simulink model "Merged_Model"  (R2020b)
settings: Solver=ode4  StartTime=0  StopTime=5000  FixedStep=0.1  MaxStep=0.1  RelTol=1e-3  EnableMultiTasking=on
values from neighbouring files (symbols this model uses):
  A_mem = 7.4    [ptoSimInputFile.m]
  A_p = V_tank_i / L_tank    (= 0.8420608)    [ptoSimInputFile.m]
  A_w = 5.56e-12    [ptoSimInputFile.m]
  angVelInit = n_shaft_ref_m    (= 50)    [ptoSimInputFile.m]
  b = b_prime / 1e3 * 1e3 * rho_f    (= 81215.9231426)    [ptoSimInputFile.m]
  C_f_i = 35    [ptoSimInputFile.m]
  D = 1.47e-9    (= 1.47e-09)    [ptoSimInputFile.m]
  eta_cp = 0.65    [ptoSimInputFile.m]
  eta_hp = 0.85    [ptoSimInputFile.m]
  eta_motor = .95    (= 0.95)    [ptoSimInputFile.m]
  J = 20*100    (= 2000)    [ptoSimInputFile.m]
  Kd = Kp*100    (= 0.001)    [ptoSimInputFile.m]
  Kd_k = Kp_k*100    (= -6.66666666667e-12)    [ptoSimInputFile.m]
  Ki = 0    [ptoSimInputFile.m]
  Ki_k = 0    [ptoSimInputFile.m]
  Kp = 1e-5    (= 1e-05)    [ptoSimInputFile.m]
  Kp_k = (-1e-13)/1.5    (= -6.66666666667e-14)    [ptoSimInputFile.m]
  L_mem = .96    (= 0.96)    [ptoSimInputFile.m]
  L_tank = 1    [ptoSimInputFile.m]
  n_par = 320    [ptoSimInputFile.m]
  n_ser = 1    [ptoSimInputFile.m]
  n_shaft_ref_m = 50    [ptoSimInputFile.m]
  nu = 8.56e-7    (= 8.56e-07)    [ptoSimInputFile.m]
  num_batches = 10*tFactor    (= 10)    [ptoSimInputFile.m]
  Omega_1_init = Q_1_init/(0.7*sqrt(2*p_h_init/rho_f))    [ptoSimInputFile.m]
  Omega_2_init = Q_2_init/(0.7*sqrt(2*p_c_init/rho_f))    [ptoSimInputFile.m]
  p_precharge = 0.9*p_lower_limit    (= 9600000)    [ptoSimInputFile.m]
  p_rated = 16e6    (= 16000000)    [ptoSimInputFile.m]
  ptosim = ptoSimClass('Non-Compressible Fluid Hydraulic')    [ptoSimInputFile.m]
  Q_cp = Q_p_des / RR_inst_des - Q_p_des    (= 0.17752896)    [ptoSimInputFile.m]
  rho_f = 1025    [ptoSimInputFile.m]
  Sc = nu/D    (= 582.31292517)    [ptoSimInputFile.m]
  thick = 7.112e-4    (= 0.0007112)    [ptoSimInputFile.m]
  V_0 = 6    [ptoSimInputFile.m]
  V_D_hpp = Q_p_des/n_shaft_ref_m    (= 0.0003945088)    [ptoSimInputFile.m]
  V_D_m = Q_2_des/n_shaft_ref_m    (= 0.000224)    [ptoSimInputFile.m]
  V_mem = A_mem * thick / 2    (= 0.00263144)    [ptoSimInputFile.m]
  V_rated = V_0*(1-(p_precharge/p_rated)^(1/1.4))    (= 1.83430127072)    [ptoSimInputFile.m]
  V_tank_i = (V_mem * n_ser * n_par * RR_tot)/(1 - RR_tot)    (= 0.8420608)    [ptoSimInputFile.m]
undefined symbols (not defined in the file or in its folder): body, constraint, pto
libraries: WECSim_Lib x5, dspswit3 x1
settings Model: Creator=mlawson  LastModifiedBy=Hayden
settings SolverCC: ZeroCrossControl=DisableAll  AlgebraicLoopSolver=LineSearch  AutoInsertRateTranBlk=on
settings DataIOCC: SaveFormat=Array  SaveOutput=off  SaveTime=off  ReturnWorkspaceOutputs=off
settings OptimizationCC: LifeSpan=inf  SimCompilerOptimization=on
settings DebuggingCC: UnderspecifiedInitializationDetection=Classic  MergeDetectMultiDrivingBlocksExec=none  SolverPrmCheckMsg=warning  AllowSymbolicDim=off  StateNameClashWarn=warning  SFUnexpectedBacktrackingDiag=warning  SFNoUnconditionalDefaultTransitionDiag=warning  ArithmeticOperatorsInVariantConditions=warning
settings HardwareCC: ProdBitPerPointer=32  ProdBitPerSizeT=32  ProdBitPerPtrDiffT=32  ProdLargestAtomicFloat=None  ProdIntDivRoundTo=Undefined  ProdEndianess=Unspecified  ProdWordSize=32  ProdHWDeviceType=32-bit Generic
settings ModelReferenceCC: PropagateSignalLabelsOutOfModel=off
settings SFSimCC: SimUseLocalCustomCode=off  CustomCodeUndefinedFunction=UseInterfaceOnly
settings RTWCC: RTWUseLocalCustomCode=off
settings CodeAppCC: StateflowObjectComments=on
settings GRTTargetCC: TargetLangStandard=C89/C90 (ANSI)
settings ConfigComp: CovMetricSettings=dw  CovSaveCumulativeToWorkspaceVar=on  CovSaveSingleToWorkspaceVar=on  CovExternalEMLEnable=off  CovSFcnEnable=off
settings SimscapeCC: SimscapeNormalizeSystem=off
settings ConfigurationSet: Description=SimMechanics 2G
settings ExplorerConfigSet: SimMechanicsOpenEditorOnUpdate=off  InternalSimMechanicsExplorerSettings="<ExplorerConfiguration><canonicalview>default</canonicalview><TilePanel><TileInfo><Tiles Columns=\"1\" Count=\"1\" Rows=\"1\"><Column Left=\"2\" Weight=\"1\"/><Column Left=\"1335\"/><Row Top=\"2\" Weight=\"1\"/><Row Top=\"911\"/><Tile Height=\"1\" Width=\"1\" X=\"0\" Y=\"0\"/></Tiles></TileInfo><SceneInfo><SceneViewer><BGColor><R>0.60000002384185791</R><G>0.60000002384185791</G><B>0.60000002384185791</B></BGColor><Camera><Position><X>365.37645888990272</X><Y>-369.82486814446582</Y><Z>359.64809521743916</Z></Position><Center><X>-6.7351450971904585</X><Y>2.2867358426280204</Y><Z>-12.463508769654169</Z></Center><Up><X>-0.40824829046386307</X><Y>0.40824829046386307</Y><Z>0.81649658092772615</Z></Up><Left>-57.820127362122818</Left><Right>57.820127362122818</Right><Bottom>-38.308817187253304</Bottom><Top>38.308817187253304</Top></Camera></SceneViewer></SceneInfo></TilePanel></ExplorerConfiguration>"

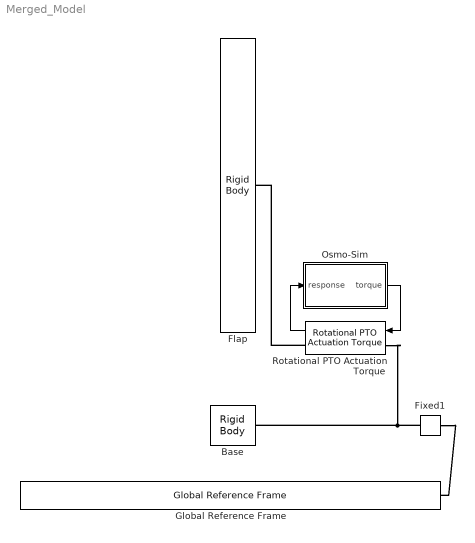
== system Merged_Model ==
  Base : WECSim_Lib/Body Elements/Rigid Body  body=body(2)
      settings: AttributesFormatString=%<body>  SourceProductName=WEC-Sim
  Fixed1 : WECSim_Lib/Constraints/Fixed  constraint=constraint(1)
      settings: AttributesFormatString=%<constraint>  SourceProductName=WEC-Sim
  Flap : WECSim_Lib/Body Elements/Rigid Body  body=body(1)
      settings: AttributesFormatString=%<body>  SourceProductName=WEC-Sim
  Global Reference Frame : WECSim_Lib/Frames/Global Reference Frame  waves=waves  simu=simu
      settings: SourceProductName=WEC-Sim
  Osmo-Sim : Subsystem
  Rotational PTO Actuation Torque : WECSim_Lib/PTOs/Rotational PTO Actuation Torque  pto=pto(1)
      settings: AttributesFormatString=%<pto>  SourceProductName=WEC-Sim
  wires:
  Rotational PTO Actuation Torque/1 -> Osmo-Sim/1(response)
  Osmo-Sim/1(torque) -> Rotational PTO Actuation Torque/1
  connections:
  Fixed1/LConn1 -- Global Reference Frame/RConn1
  Fixed1/RConn1 -- Rotational PTO Actuation Torque/LConn1 -- Base/RConn1
  Rotational PTO Actuation Torque/RConn1 -- Flap/RConn1

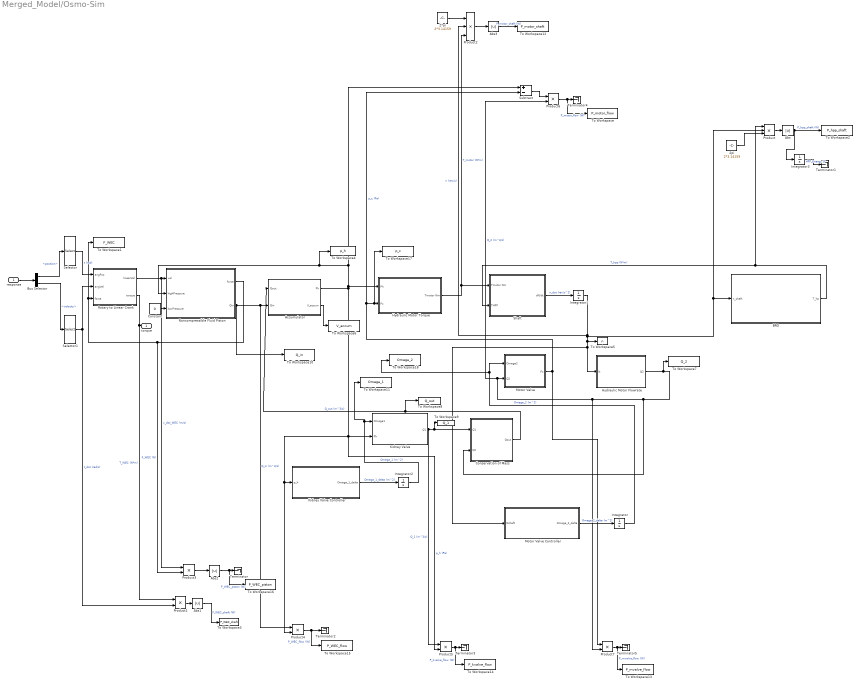
== system Merged_Model/Osmo-Sim ==
  response : Inport
  2*pi : Constant  Value=2*3.14159
  2pi : Constant  Value=2*3.14159  OutDataTypeStr=Inherit: Inherit via back propagation
  Abs{,1..3} (4 alike) : Abs
  Accumulator : Subsystem
  BRO : Subsystem
  Bus Selector : BusSelector  OutputSignals=position,velocity
  Conservation of Mass : Subsystem
  Constant : Constant  Value=0
  Hydraulic Motor Flowrate : Subsystem
  Hydraulic Motor Torque : Subsystem
  Integrator : Integrator  InitialCondition=Omega_2_init
  Integrator1 : Integrator  InitialCondition=angVelInit
  Integrator2 : Integrator  InitialCondition=Omega_1_init
  Integrator3 : Integrator
  Kidney Valve : Subsystem
  Kidney Valve Controller : Subsystem
  Motor Valve : Subsystem
  Motor Valve Controller : Subsystem
  Noncompressible Fluid Piston : Subsystem  mask{ptosim=ptosim.pistonNCF(1)}
      mask prompts: ptosim "Piston Name:"
      mask init:
      | if exist ('ptosim','var')
      |     h = [gcb '/To Workspace'];
      |     responseName = ['pistonNCF' num2str(ptosim.number) '_out'];
      |     set_param(h,'VariableName',responseName);
      |     if ischar(ptosim.topA)==1 ...
      |       || ischar(ptosim.botA)==1
      |          error('One of the piston variables is undefined. For example, ptosim.pistonNCF.variableName')
      |     end
      | end
      | clear h responseName
  Product : Product  Inputs=3
  Product{1,3..7} (6 alike) : Product
  Product2 : Product  Inputs=3
  Rotary to Linear Crank : Subsystem  AncestorBlock=PTOSim_Lib/Motion Conversion/Rotary to Linear Crank  mask{ptosim=ptosim.motionMechanism(1)}
      mask prompts: ptosim "Crank Name:"
      mask init:
      | if exist('ptosim','var')
      |     h = [gcb '/To Workspace'];
      |     responseName = ['motionMechanism' num2str(ptosim.number) '_out'];
      |     set_param(h,'VariableName',responseName);
      |     if ischar(ptosim.crank)==1 ...
      |             || ischar(ptosim.rodLength)==1 ...
      |             || ischar(ptosim.offset)==1 ...
      |             error('One of the rotary to linear crank variables is undefined. For example, ptosim.motionMechanism.variableName')
      |     end
      | end
      | clear h responseName
  Selector : Selector  InputPortWidth=6  IndexOptions=Index vector (dialog)  Indices=5  OutputSizes=1
  Selector1 : Selector  InputPortWidth=6  IndexOptions=Index vector (dialog)  Indices=5  OutputSizes=1
  Shaft : Subsystem
  Subtract : Sum  Inputs=+-
  Terminator{,1..5} (6 alike) : Terminator
  To Workspace : ToWorkspace  VariableName=P_motor_flow  SaveFormat=Timeseries  SampleTime=-1
  To Workspace1 : ToWorkspace  VariableName=F_WEC  SaveFormat=Timeseries  SampleTime=-1
  To Workspace10 : ToWorkspace  VariableName=Q_in  SaveFormat=Timeseries  SampleTime=-1
  To Workspace11 : ToWorkspace  VariableName=Omega_1  SaveFormat=Timeseries  SampleTime=-1
  To Workspace12 : ToWorkspace  VariableName=P_motor_shaft  SaveFormat=Timeseries  SampleTime=-1
  To Workspace13 : ToWorkspace  VariableName=P_mvalve_flow  SaveFormat=Timeseries  SampleTime=-1
  To Workspace14 : ToWorkspace  VariableName=P_kvalve_flow  SaveFormat=Timeseries  SampleTime=-1
  To Workspace15 : ToWorkspace  VariableName=P_WEC_flow  SaveFormat=Timeseries  SampleTime=-1
  To Workspace16 : ToWorkspace  VariableName=P_WEC_piston  SaveFormat=Timeseries  SampleTime=-1
  To Workspace17 : ToWorkspace  VariableName=p_c  SaveFormat=Timeseries  SampleTime=-1
  To Workspace18 : ToWorkspace  VariableName=Omega_2  SaveFormat=Timeseries  SampleTime=-1
  To Workspace2 : ToWorkspace  VariableName=P_hpp_shaft  SaveFormat=Timeseries  SampleTime=-1
  To Workspace3 : ToWorkspace  VariableName=P_WEC_shaft  SaveFormat=Timeseries  SampleTime=-1
  To Workspace4 : ToWorkspace  VariableName=p_h  SaveFormat=Timeseries  SampleTime=-1
  To Workspace5 : ToWorkspace  VariableName=n  SaveFormat=Timeseries  SampleTime=-1
  To Workspace6 : ToWorkspace  VariableName=V_accum  SaveFormat=Timeseries  SampleTime=-1
  To Workspace7 : ToWorkspace  VariableName=Q_2  SaveFormat=Timeseries  SampleTime=-1
  To Workspace8 : ToWorkspace  VariableName=Q_out  SaveFormat=Timeseries  SampleTime=-1
  To Workspace9 : ToWorkspace  VariableName=Q_1  SaveFormat=Timeseries  SampleTime=-1
  torque : Outport  VectorParamsAs1DForOutWhenUnconnected=off
  wires:
  response/1 -> Bus Selector/1
  Bus Selector/1 -> Selector/1  "<position>"
  Bus Selector/2 -> Selector1/1  "<velocity>"
  Rotary to Linear Crank/2(torque) -> Product1/1, torque/1  "T_WEC (N*m)"
  Selector/1 -> Rotary to Linear Crank/1(angPos)  "t (rad)"
  Selector1/1 -> Rotary to Linear Crank/2(angVel), Product1/2  "t_dot (rad/s)"
  Rotary to Linear Crank/1(linearVel) -> Product3/1, Noncompressible Fluid Piston/1(vel)  "x_dot_WEC (m/s)"
  Noncompressible Fluid Piston/1(force) -> Product3/2, To Workspace1/1, Rotary to Linear Crank/3(force)  "F_WEC (N)"
  Constant/1 -> Noncompressible Fluid Piston/3(lowPressure)
  Accumulator/1(Ph) -> Subtract/1, Noncompressible Fluid Piston/2(highPressure), To Workspace4/1, Hydraulic Motor Torque/1(Ph), Product5/2, Product4/2, Kidney Valve Controller/1(p_h), Kidney Valve/2(Ph)  "p_h (Pa)"
  Noncompressible Fluid Piston/2(Qin) -> To Workspace10/1, Product4/1, Accumulator/2(Qin)  "Q_in (m^3/s)"
  Motor Valve/1(Pc) -> Subtract/2, To Workspace17/1, Hydraulic Motor Torque/2(Pc), Product7/1  "p_c (Pa)"
  BRO/1(T_hp) -> Shaft/2(THPP), Product/1  "T_hpp (N*m)"
  Hydraulic Motor Torque/1(Tmotor Nm) -> Shaft/1(Tmotor Nm), Product2/3  "T_motor (N*m)"
  Integrator1/1 -> BRO/1(n_shaft), Product/2, Hydraulic Motor Flowrate/1(N), Motor Valve Controller/1(Nshaft), To Workspace5/1, Product2/2  "n (rev/s)"
  Shaft/1(dN/dt) -> Integrator1/1  "n_dot (rev/s^2)"
  Kidney Valve/1(Q1) -> Product5/1, Conservation of Mass/1(Q1), To Workspace9/1  "Q_1 (m^3/s)"
  Conservation of Mass/1(Qout) -> To Workspace8/1, Accumulator/1(Qout)  "Q_out (m^3/s)"
  Product/1 -> Abs/1
  Product1/1 -> Abs1/1
  2pi/1 -> Product/3
  Abs/1 -> Integrator3/1, To Workspace2/1  "P_hpp_shaft (W)"
  Abs1/1 -> To Workspace3/1  "P_WEC_shaft (W)"
  Hydraulic Motor Flowrate/1(Q2) -> To Workspace7/1, Conservation of Mass/2(Q2), Product7/2, Motor Valve/2(Q2), Product6/2  "Q_2 (m^3/s)"
  Motor Valve Controller/1(Omega_2_delta) -> Integrator/1  "Omega_2_delta (m^2)"
  Integrator/1 -> To Workspace18/1, Motor Valve/1(Omega2)  "Omega_2 (m^2)"
  Accumulator/2(V_accum) -> To Workspace6/1
  Kidney Valve Controller/1(Omega_1_delta) -> Integrator2/1  "Omega_1_delta (m^2)"
  Integrator2/1 -> To Workspace11/1, Kidney Valve/1(Omega1)  "Omega_1 (m^2)"
  2*pi/1 -> Product2/1
  Product3/1 -> Abs2/1
  Abs2/1 -> To Workspace16/1, Terminator/1  "P_WEC_piston (W)"
  Integrator3/1 -> Terminator1/1  "HPP_Energy (J)"
  Product2/1 -> Abs3/1
  Abs3/1 -> To Workspace12/1  "P_motor_shaft (W)"
  Product4/1 -> To Workspace15/1, Terminator2/1  "P_WEC_flow (W)"
  Product5/1 -> To Workspace14/1, Terminator3/1  "P_kvalve_flow (W)"
  Subtract/1 -> Product6/1
  Product6/1 -> To Workspace/1, Terminator4/1  "P_motor_flow (W)"
  Product7/1 -> To Workspace13/1, Terminator5/1  "P_mvalve_flow (W)"

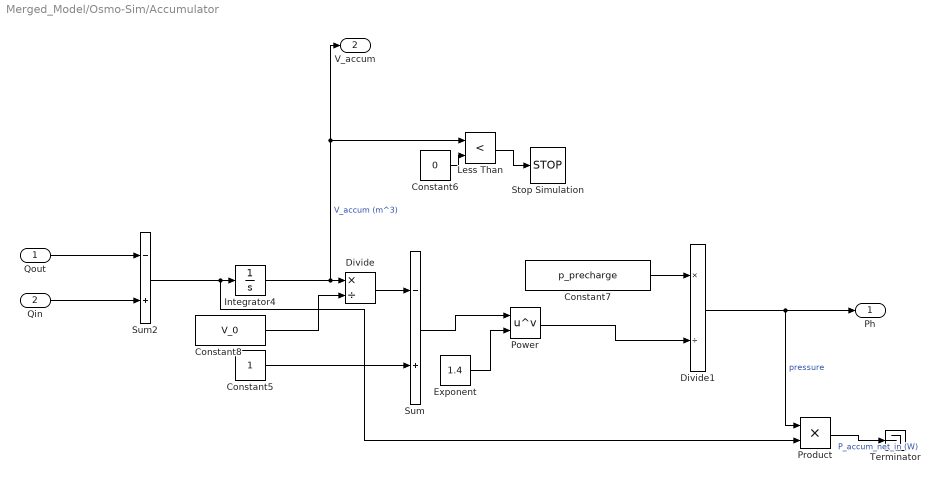
== system Merged_Model/Osmo-Sim/Accumulator ==
  Qout : Inport
  Qin : Inport  Port=2
  Constant5 : Constant
  Constant6 : Constant  Value=0
  Constant7 : Constant  Value=p_precharge
  Constant8 : Constant  Value=V_0
  Divide : Product  Inputs=*/
  Divide1 : Product  Inputs=*/
  Exponent : Constant  Value=1.4
  Integrator4 : Integrator  InitialCondition=V_rated
  Less Than : RelationalOperator  Operator=<  OutDataTypeStr=boolean  RndMeth=Simplest
  Power : Math  Operator=pow  SaturateOnIntegerOverflow=on
  Product : Product
  Stop Simulation : Stop
  Sum : Sum  Inputs=-+
  Sum2 : Sum  Inputs=-+
  Terminator : Terminator
  Ph : Outport
  V_accum : Outport  Port=2
  wires:
  Constant8/1 -> Divide/2
  Qout/1 -> Sum2/1
  Power/1 -> Divide1/2
  Less Than/1 -> Stop Simulation/1
  Integrator4/1 -> V_accum/1, Less Than/1, Divide/1  "V_accum (m^3)"
  Constant7/1 -> Divide1/1
  Divide1/1 -> Product/1, Ph/1  "pressure"
  Divide/1 -> Sum/1
  Constant5/1 -> Sum/2
  Qin/1 -> Sum2/2
  Constant6/1 -> Less Than/2
  Sum2/1 -> Product/2, Integrator4/1
  Exponent/1 -> Power/2
  Sum/1 -> Power/1
  Product/1 -> Terminator/1  "P_accum_net_in (W)"

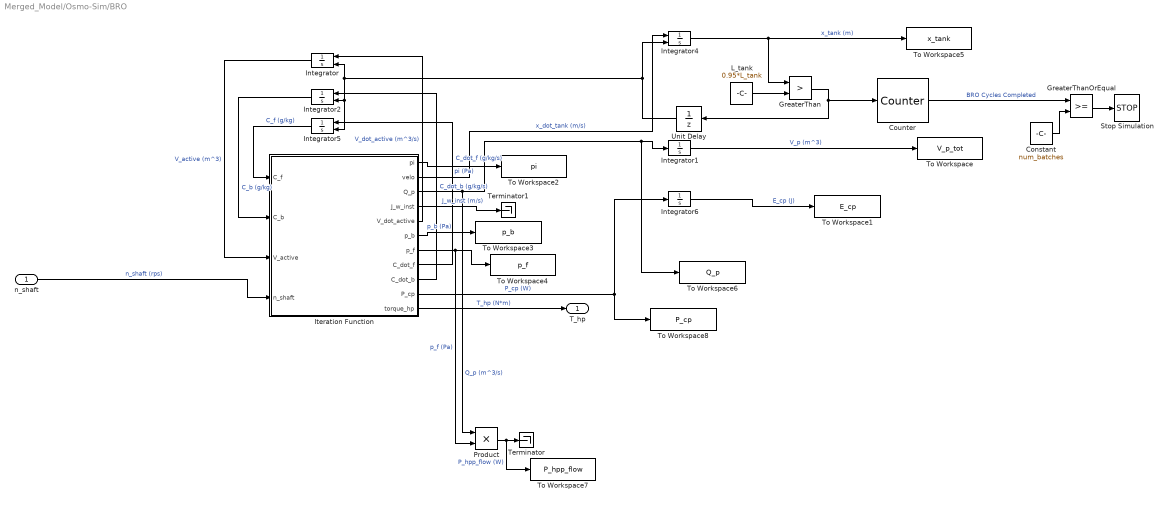
== system Merged_Model/Osmo-Sim/BRO ==
  n_shaft : Inport
  Constant : Constant  Value=num_batches
  Counter : dspswit3/Counter  Direction=Up  CountEvent=Rising edge  CounterSize=User defined  MaxCount=255  InitialCount=0  Output=Count  HitValue=32  ResetInput=off  SamplesPerFrame=1  Ts=1  CntDtype=double  HitDtype=Logical
  GreaterThan : RelationalOperator  Operator=>  OutDataTypeStr=boolean  RndMeth=Simplest
  GreaterThanOrEqual : RelationalOperator  OutDataTypeStr=boolean  RndMeth=Simplest
  Integrator : Integrator  ExternalReset=rising  InitialCondition=V_tank_i
  Integrator1 : Integrator
  Integrator2 : Integrator  ExternalReset=rising  InitialCondition=C_f_i
  Integrator4 : Integrator  ExternalReset=rising
  Integrator5 : Integrator  ExternalReset=rising  InitialCondition=C_f_i
  Integrator6 : Integrator
  Iteration Function : MATLAB Function  TreatAsAtomicUnit=on
  L_tank : Constant  Value=0.95*L_tank
  Product : Product
  Stop Simulation : Stop
  Terminator : Terminator
  Terminator1 : Terminator
  To Workspace : ToWorkspace  VariableName=V_p_tot  SaveFormat=Timeseries  SampleTime=-1
  To Workspace1 : ToWorkspace  VariableName=E_cp  SaveFormat=Timeseries  SampleTime=-1
  To Workspace2 : ToWorkspace  VariableName=pi  SaveFormat=Timeseries  SampleTime=-1
  To Workspace3 : ToWorkspace  VariableName=p_b  SaveFormat=Timeseries  SampleTime=-1
  To Workspace4 : ToWorkspace  VariableName=p_f  SaveFormat=Timeseries  SampleTime=-1
  To Workspace5 : ToWorkspace  VariableName=x_tank  SaveFormat=Timeseries  SampleTime=-1
  To Workspace6 : ToWorkspace  VariableName=Q_p  SaveFormat=Timeseries  SampleTime=-1
  To Workspace7 : ToWorkspace  VariableName=P_hpp_flow  SaveFormat=Timeseries  SampleTime=-1
  To Workspace8 : ToWorkspace  VariableName=P_cp  SaveFormat=Timeseries  SampleTime=-1
  Unit Delay : UnitDelay  SampleTime=-1  HasFrameUpgradeWarning=on
  T_hp : Outport
  wires:
  Integrator2/1 -> Iteration Function/2(C_b)  "C_b (g/kg)"
  Iteration Function/7(p_f) -> Product/2, To Workspace4/1  "p_f (Pa)"
  Iteration Function/5(V_dot_active) -> Integrator/1  "V_dot_active (m^3/s)"
  GreaterThan/1 -> Counter/1, Unit Delay/1
  Iteration Function/8(C_dot_f) -> Integrator5/1  "C_dot_f (g/kg/s)"
  Integrator1/1 -> To Workspace/1  "V_p (m^3)"
  L_tank/1 -> GreaterThan/2
  Integrator/1 -> Iteration Function/3(V_active)  "V_active (m^3)"
  Iteration Function/3(Q_p) -> To Workspace6/1, Integrator1/1, Product/1  "Q_p (m^3/s)"
  Iteration Function/9(C_dot_b) -> Integrator2/1  "C_dot_b (g/kg/s)"
  Integrator4/1 -> To Workspace5/1, GreaterThan/1  "x_tank (m)"
  Iteration Function/10(P_cp) -> Integrator6/1, To Workspace8/1  "P_cp (W)"
  Iteration Function/2(velo) -> Integrator4/1  "x_dot_tank (m/s)"
  Integrator5/1 -> Iteration Function/1(C_f)  "C_f (g/kg)"
  Iteration Function/6(p_b) -> To Workspace3/1  "p_b (Pa)"
  Iteration Function/4(J_w_inst) -> Terminator1/1  "J_w_inst (m/s)"
  Iteration Function/1(pi) -> To Workspace2/1  "pi (Pa)"
  Integrator6/1 -> To Workspace1/1  "E_cp (J)"
  Unit Delay/1 -> Integrator4/2, Integrator5/2, Integrator2/2, Integrator/2
  Counter/1 -> GreaterThanOrEqual/1  "BRO Cycles Completed"
  Constant/1 -> GreaterThanOrEqual/2
  GreaterThanOrEqual/1 -> Stop Simulation/1
  Iteration Function/11(torque_hp) -> T_hp/1  "T_hp (N*m)"
  n_shaft/1 -> Iteration Function/4(n_shaft)  "n_shaft (rps)"
  Product/1 -> To Workspace7/1, Terminator/1  "P_hpp_flow (W)"

== system Merged_Model/Osmo-Sim/Conservation of Mass ==
  Q1 : Inport
  Q2 : Inport  Port=2
  Add1 : Sum
  Qout : Outport
  wires:
  Add1/1 -> Qout/1
  Q2/1 -> Add1/1
  Q1/1 -> Add1/2

== system Merged_Model/Osmo-Sim/Hydraulic Motor Flowrate ==
  N : Inport
  Product2 : Product
  V_D_m : Constant  Value=V_D_m
  Q2 : Outport
  wires:
  Product2/1 -> Q2/1  "Q2"
  V_D_m/1 -> Product2/2
  N/1 -> Product2/1

== system Merged_Model/Osmo-Sim/Hydraulic Motor Torque ==
  Ph : Inport
  Pc : Inport  Port=2
  2pi : Constant  Value=2*3.14159
  Eta Motor : Constant  Value=eta_motor
  Product2 : Product  Inputs=***/
  Sum2 : Sum  Inputs=+-
  Vdm : Constant  Value=V_D_m
  Tmotor Nm : Outport
  wires:
  Eta Motor/1 -> Product2/3
  Ph/1 -> Sum2/1
  Product2/1 -> Tmotor Nm/1
  Vdm/1 -> Product2/2
  Sum2/1 -> Product2/1
  Pc/1 -> Sum2/2
  2pi/1 -> Product2/4

== system Merged_Model/Osmo-Sim/Kidney Valve ==
  note: Q1
  Omega1 : Inport
  Ph : Inport  Port=2
  Cf1 : Constant  Value=0.7
  Divide1 : Product  Inputs=***
  Divide2 : Product  Inputs=*/
  Gain1 : Gain  Gain=2
  Square Root1 : Sqrt  SaturateOnIntegerOverflow=on
  rho (kg/m^3) : Constant  Value=1025
  Q1 : Outport
  wires:
  Divide2/1 -> Square Root1/1
  Cf1/1 -> Divide1/1
  Square Root1/1 -> Divide1/3
  rho (kg/m^3)/1 -> Divide2/2
  Gain1/1 -> Divide2/1
  Divide1/1 -> Q1/1
  Ph/1 -> Gain1/1
  Omega1/1 -> Divide1/2

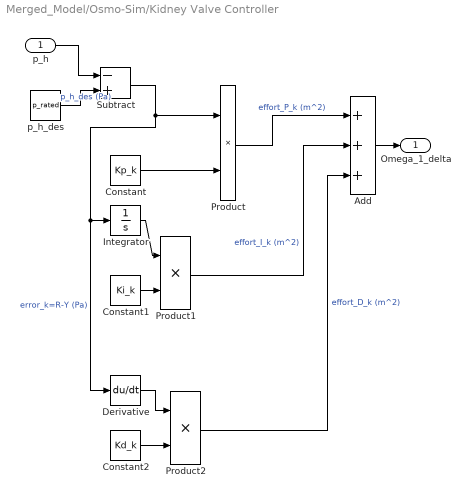
== system Merged_Model/Osmo-Sim/Kidney Valve Controller ==
  p_h : Inport
  Add : Sum  Inputs=+++
  Constant : Constant  Value=Kp_k
  Constant1 : Constant  Value=Ki_k
  Constant2 : Constant  Value=Kd_k
  Derivative : Derivative
  Integrator : Integrator
  Product : Product
  Product1 : Product
  Product2 : Product
  Subtract : Sum  Inputs=-+
  p_h_des : Constant  Value=p_rated
  Omega_1_delta : Outport
  wires:
  p_h/1 -> Subtract/1
  p_h_des/1 -> Subtract/2  "p_h_des (Pa)"
  Subtract/1 -> Product/1, Derivative/1, Integrator/1  "error_k=R-Y (Pa)"
  Integrator/1 -> Product1/1
  Constant1/1 -> Product1/2
  Constant/1 -> Product/2
  Product/1 -> Add/1  "effort_P_k (m^2)"
  Product1/1 -> Add/2  "effort_I_k (m^2)"
  Add/1 -> Omega_1_delta/1
  Constant2/1 -> Product2/2
  Derivative/1 -> Product2/1
  Product2/1 -> Add/3  "effort_D_k (m^2)"

== system Merged_Model/Osmo-Sim/Motor Valve ==
  Omega2 : Inport
  Q2 : Inport  Port=2
  Cf1 : Constant  Value=0.7
  Constant : Constant  Value=2
  Product : Product  Inputs=**/
  Product2 : Product  Inputs=*//
  Square : Math  Operator=square  SaturateOnIntegerOverflow=on
  rho (kg/m^3)1 : Constant  Value=1025
  Pc : Outport
  wires:
  Product/1 -> Pc/1
  Cf1/1 -> Product2/2
  Product2/1 -> Square/1
  Square/1 -> Product/1
  rho (kg/m^3)1/1 -> Product/2
  Constant/1 -> Product/3
  Omega2/1 -> Product2/3
  Q2/1 -> Product2/1

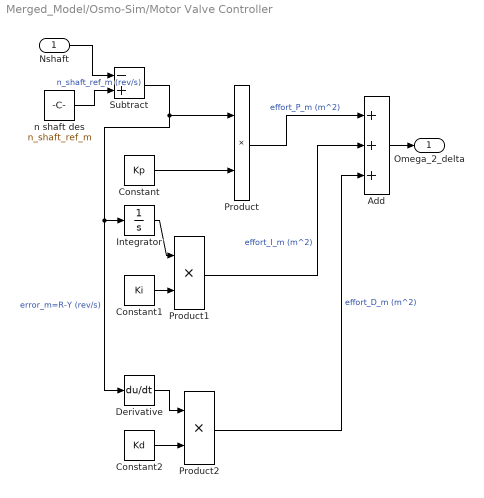
== system Merged_Model/Osmo-Sim/Motor Valve Controller ==
  Nshaft : Inport
  Add : Sum  Inputs=+++
  Constant : Constant  Value=Kp
  Constant1 : Constant  Value=Ki
  Constant2 : Constant  Value=Kd
  Derivative : Derivative
  Integrator : Integrator
  Product : Product
  Product1 : Product
  Product2 : Product
  Subtract : Sum  Inputs=-+
  n shaft des : Constant  Value=n_shaft_ref_m
  Omega_2_delta : Outport
  wires:
  Nshaft/1 -> Subtract/1
  n shaft des/1 -> Subtract/2  "n_shaft_ref_m (rev/s)"
  Subtract/1 -> Product/1, Derivative/1, Integrator/1  "error_m=R-Y (rev/s)"
  Integrator/1 -> Product1/1
  Constant1/1 -> Product1/2
  Constant/1 -> Product/2
  Product/1 -> Add/1  "effort_P_m (m^2)"
  Product1/1 -> Add/2  "effort_I_m (m^2)"
  Add/1 -> Omega_2_delta/1
  Constant2/1 -> Product2/2
  Derivative/1 -> Product2/1
  Product2/1 -> Add/3  "effort_D_m (m^2)"

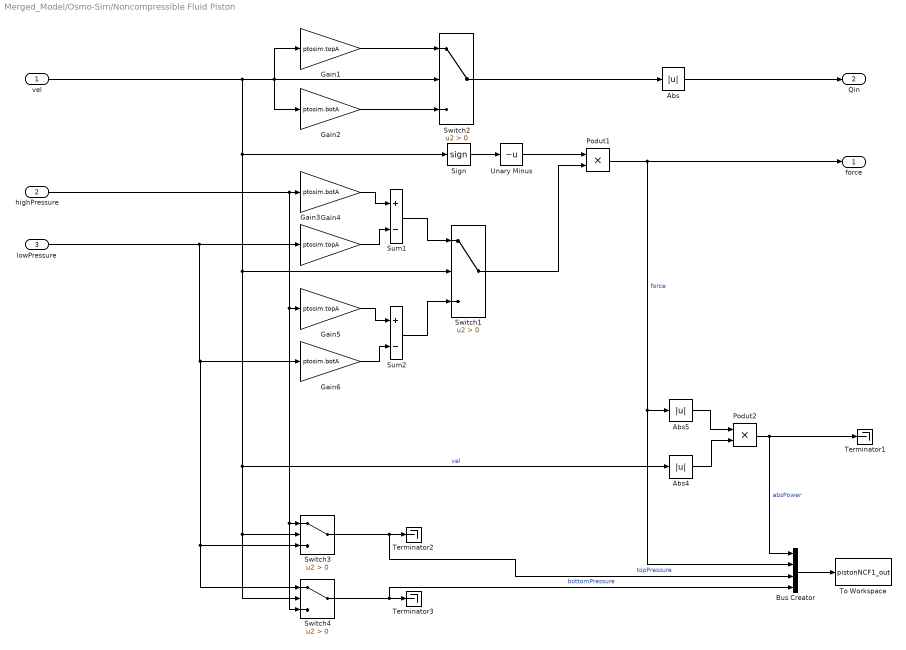
== system Merged_Model/Osmo-Sim/Noncompressible Fluid Piston ==
  vel : Inport
  highPressure : Inport  Port=2
  lowPressure : Inport  Port=3
  Abs : Abs
  Abs4 : Abs
  Abs5 : Abs
  Bus Creator : BusCreator  Inputs=4
  Gain1 : Gain  Gain=ptosim.topA
  Gain2 : Gain  Gain=ptosim.botA
  Gain3 : Gain  Gain=ptosim.topA
  Gain4 : Gain  Gain=ptosim.botA
  Gain5 : Gain  Gain=ptosim.topA
  Gain6 : Gain  Gain=ptosim.botA
  Podut1 : Product  RndMeth=Zero
  Podut2 : Product  RndMeth=Zero
  Sign : Signum
  Sum1 : Sum  Inputs=+-
  Sum2 : Sum  Inputs=+-
  Switch{1..4} (4 alike) : Switch  Criteria=u2 > Threshold
  Terminator1 : Terminator
  Terminator2 : Terminator
  Terminator3 : Terminator
  To Workspace : ToWorkspace  VariableName=pistonNCF1_out  SaveFormat=Structure With Time  SampleTime=-1
      settings: Decimation=round(simu.dtOut/simu.dt,0)
  Unary Minus : UnaryMinus
  force : Outport
  Qin : Outport  Port=2
  wires:
  Bus Creator/1 -> To Workspace/1
  Switch4/1 -> Terminator3/1, Bus Creator/4  "bottomPressure"
  Switch3/1 -> Terminator2/1, Bus Creator/3  "topPressure"
  Switch1/1 -> Podut1/2
  Unary Minus/1 -> Podut1/1
  Sign/1 -> Unary Minus/1
  Sum2/1 -> Switch1/3
  Gain6/1 -> Sum2/2
  Gain5/1 -> Sum2/1
  lowPressure/1 -> Gain3/1, Gain6/1, Switch3/3, Switch4/1
  Gain3/1 -> Sum1/2
  Gain4/1 -> Sum1/1
  Podut1/1 -> Abs5/1, Bus Creator/2, force/1  "force"
  Sum1/1 -> Switch1/1
  Gain2/1 -> Switch2/3
  Gain1/1 -> Switch2/1
  Abs4/1 -> Podut2/2
  Abs5/1 -> Podut2/1
  Podut2/1 -> Terminator1/1, Bus Creator/1  "absPower"
  vel/1 -> Gain1/1, Switch2/2, Gain2/1, Sign/1, Abs4/1, Switch3/2, Switch4/2, Switch1/2  "vel"
  highPressure/1 -> Gain5/1, Switch4/3, Switch3/1, Gain4/1
  Switch2/1 -> Abs/1
  Abs/1 -> Qin/1

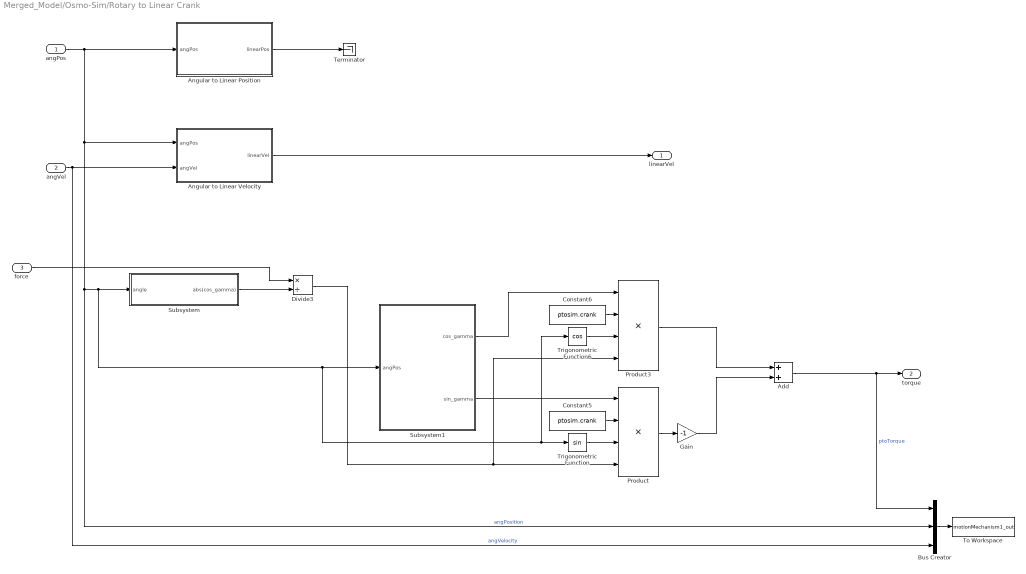
== system Merged_Model/Osmo-Sim/Rotary to Linear Crank ==
  angPos : Inport
  angVel : Inport  Port=2
  force : Inport  Port=3
  Add : Sum
  Angular to Linear Position : Subsystem
  Angular to Linear Velocity : Subsystem
  Bus Creator : BusCreator  Inputs=3
  Constant5 : Constant  Value=ptosim.crank
  Constant6 : Constant  Value=ptosim.crank
  Divide3 : Product  Inputs=*/
  Gain : Gain  Gain=-1
  Product : Product  Inputs=4
  Product3 : Product  Inputs=4
  Subsystem : Subsystem
  Subsystem1 : Subsystem  AncestorBlock=PTOSim_Lib/Motion Conversion/Rotary to Linear Adjustable Rod/Subsystem
  Terminator : Terminator
  To Workspace : ToWorkspace  VariableName=motionMechanism1_out  SaveFormat=Structure With Time  SampleTime=-1
      settings: Decimation=round(simu.dtOut/simu.dt,0)
  Trigonometric Function : Trigonometry
  Trigonometric Function6 : Trigonometry  Operator=cos
  linearVel : Outport
  torque : Outport  Port=2
  wires:
  Product/1 -> Gain/1
  Constant5/1 -> Product/2
  Trigonometric Function/1 -> Product/3
  angPos/1 -> Angular to Linear Position/1(angPos), Bus Creator/2, Subsystem/1(angle), Trigonometric Function6/1, Trigonometric Function/1, Subsystem1/1(angPos), Angular to Linear Velocity/1(angPos)  "angPosition"
  Subsystem1/2(sin_gamma) -> Product/1
  Product3/1 -> Add/1
  Gain/1 -> Add/2
  Divide3/1 -> Product3/4, Product/4
  Constant6/1 -> Product3/2
  Subsystem1/1(cos_gamma) -> Product3/1
  Trigonometric Function6/1 -> Product3/3
  force/1 -> Divide3/1
  Subsystem/1(abs(cos_gamma)) -> Divide3/2
  Bus Creator/1 -> To Workspace/1
  Add/1 -> torque/1, Bus Creator/1  "ptoTorque"
  Angular to Linear Velocity/1(linearVel) -> linearVel/1
  angVel/1 -> Angular to Linear Velocity/2(angVel), Bus Creator/3  "angVelocity"
  Angular to Linear Position/1(linearPos) -> Terminator/1

== system Merged_Model/Osmo-Sim/Shaft ==
  Tmotor Nm : Inport
  THPP : Inport  Port=2
  Constant4 : Constant  Value=2*pi
  Constant5 : Constant  Value=J
  Divide2 : Product  Inputs=*//
  Sum1 : Sum
  dN/dt : Outport
  wires:
  Constant4/1 -> Divide2/3
  Sum1/1 -> Divide2/1
  THPP/1 -> Sum1/2
  Constant5/1 -> Divide2/2
  Divide2/1 -> dN/dt/1  "dN/dt"
  Tmotor Nm/1 -> Sum1/1

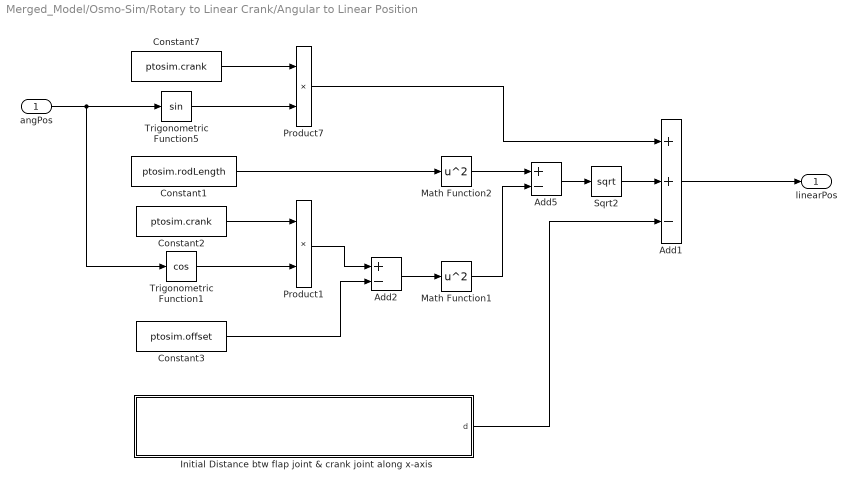
== system Merged_Model/Osmo-Sim/Rotary to Linear Crank/Angular to Linear Position ==
  angPos : Inport
  Add1 : Sum  Inputs=++-
  Add2 : Sum  Inputs=+-
  Add5 : Sum  Inputs=+-
  Constant1 : Constant  Value=ptosim.rodLength
  Constant2 : Constant  Value=ptosim.crank
  Constant3 : Constant  Value=ptosim.offset
  Constant7 : Constant  Value=ptosim.crank
  Initial Distance btw flap joint & crank joint along x-axis : Subsystem
  Math Function1 : Math  Operator=square  SignedPower=on  SaturateOnIntegerOverflow=on
  Math Function2 : Math  Operator=square  SignedPower=on  SaturateOnIntegerOverflow=on
  Product1 : Product  Inputs=**
  Product7 : Product  Inputs=**
  Sqrt2 : Sqrt  SaturateOnIntegerOverflow=on
  Trigonometric Function1 : Trigonometry  Operator=cos
  Trigonometric Function5 : Trigonometry
  linearPos : Outport
  wires:
  Math Function2/1 -> Add5/1
  Add1/1 -> linearPos/1
  Product7/1 -> Add1/1
  Sqrt2/1 -> Add1/2
  Math Function1/1 -> Add5/2
  Constant1/1 -> Math Function2/1
  Initial Distance btw flap joint & crank joint along x-axis/1(d) -> Add1/3
  Constant7/1 -> Product7/1
  Constant3/1 -> Add2/2
  Product1/1 -> Add2/1
  Trigonometric Function1/1 -> Product1/2
  Constant2/1 -> Product1/1
  Add5/1 -> Sqrt2/1
  Trigonometric Function5/1 -> Product7/2
  Add2/1 -> Math Function1/1
  angPos/1 -> Trigonometric Function5/1, Trigonometric Function1/1

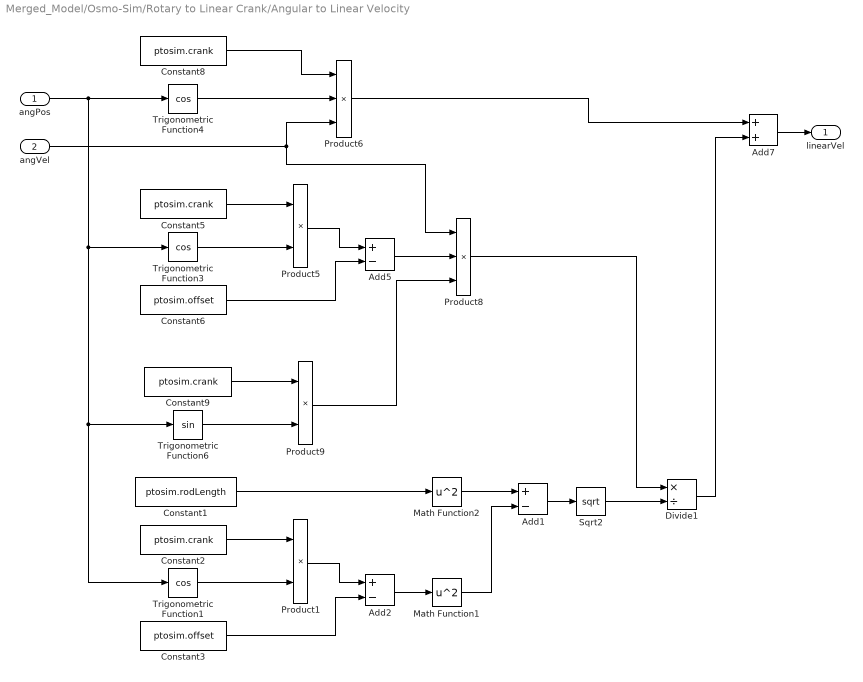
== system Merged_Model/Osmo-Sim/Rotary to Linear Crank/Angular to Linear Velocity ==
  angPos : Inport
  angVel : Inport  Port=2
  Add1 : Sum  Inputs=+-
  Add2 : Sum  Inputs=+-
  Add5 : Sum  Inputs=+-
  Add7 : Sum
  Constant1 : Constant  Value=ptosim.rodLength
  Constant{2,5,8..9} (4 alike) : Constant  Value=ptosim.crank
  Constant3 : Constant  Value=ptosim.offset
  Constant6 : Constant  Value=ptosim.offset
  Divide1 : Product  Inputs=*/
  Math Function1 : Math  Operator=square  SignedPower=on  SaturateOnIntegerOverflow=on
  Math Function2 : Math  Operator=square  SignedPower=on  SaturateOnIntegerOverflow=on
  Product1 : Product  Inputs=**
  Product5 : Product  Inputs=**
  Product6 : Product  Inputs=***
  Product8 : Product  Inputs=***
  Product9 : Product  Inputs=**
  Sqrt2 : Sqrt  SaturateOnIntegerOverflow=on
  Trigonometric Function1 : Trigonometry  Operator=cos
  Trigonometric Function3 : Trigonometry  Operator=cos
  Trigonometric Function4 : Trigonometry  Operator=cos
  Trigonometric Function6 : Trigonometry
  linearVel : Outport
  wires:
  Math Function2/1 -> Add1/1
  Divide1/1 -> Add7/2
  Product8/1 -> Divide1/1
  Sqrt2/1 -> Divide1/2
  Math Function1/1 -> Add1/2
  Constant1/1 -> Math Function2/1
  Constant3/1 -> Add2/2
  Product1/1 -> Add2/1
  Trigonometric Function1/1 -> Product1/2
  Constant2/1 -> Product1/1
  Add1/1 -> Sqrt2/1
  Add2/1 -> Math Function1/1
  angPos/1 -> Trigonometric Function4/1, Trigonometric Function3/1, Trigonometric Function6/1, Trigonometric Function1/1
  Product9/1 -> Product8/3
  Add5/1 -> Product8/2
  angVel/1 -> Product6/3, Product8/1
  Trigonometric Function6/1 -> Product9/2
  Constant9/1 -> Product9/1
  Constant6/1 -> Add5/2
  Product5/1 -> Add5/1
  Trigonometric Function3/1 -> Product5/2
  Constant5/1 -> Product5/1
  Product6/1 -> Add7/1
  Constant8/1 -> Product6/1
  Trigonometric Function4/1 -> Product6/2
  Add7/1 -> linearVel/1

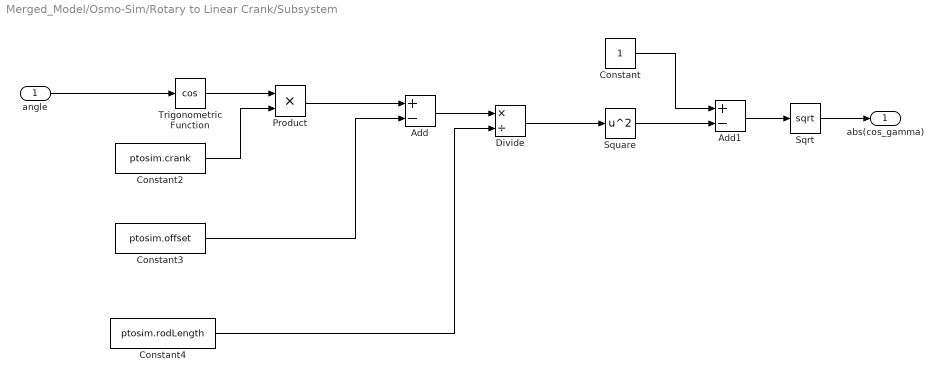
== system Merged_Model/Osmo-Sim/Rotary to Linear Crank/Subsystem ==
  angle : Inport
  Add : Sum  Inputs=+-
  Add1 : Sum  Inputs=+-
  Constant : Constant
  Constant2 : Constant  Value=ptosim.crank
  Constant3 : Constant  Value=ptosim.offset
  Constant4 : Constant  Value=ptosim.rodLength
  Divide : Product  Inputs=*/
  Product : Product
  Sqrt : Sqrt  SaturateOnIntegerOverflow=on
  Square : Math  Operator=square  SignedPower=on  SaturateOnIntegerOverflow=on
  Trigonometric Function : Trigonometry  Operator=cos
  abs(cos_gamma) : Outport
  wires:
  Sqrt/1 -> abs(cos_gamma)/1
  Constant/1 -> Add1/1
  Add1/1 -> Sqrt/1
  Square/1 -> Add1/2
  Divide/1 -> Square/1
  Constant4/1 -> Divide/2
  Add/1 -> Divide/1
  Constant3/1 -> Add/2
  Product/1 -> Add/1
  Constant2/1 -> Product/2
  Trigonometric Function/1 -> Product/1
  angle/1 -> Trigonometric Function/1

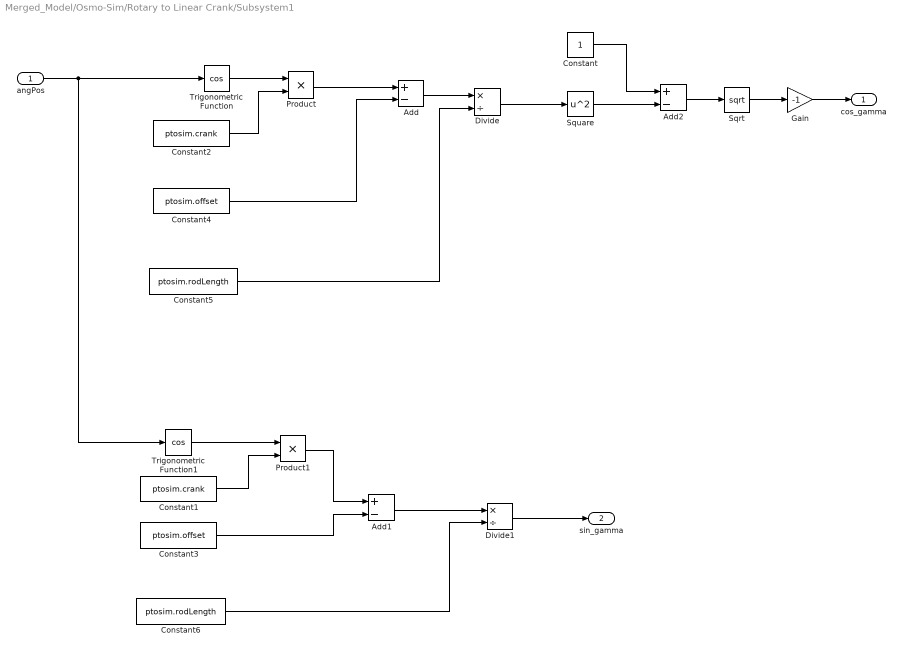
== system Merged_Model/Osmo-Sim/Rotary to Linear Crank/Subsystem1 ==
  angPos : Inport
  Add : Sum  Inputs=+-
  Add1 : Sum  Inputs=+-
  Add2 : Sum  Inputs=+-
  Constant : Constant
  Constant1 : Constant  Value=ptosim.crank
  Constant2 : Constant  Value=ptosim.crank
  Constant3 : Constant  Value=ptosim.offset
  Constant4 : Constant  Value=ptosim.offset
  Constant5 : Constant  Value=ptosim.rodLength
  Constant6 : Constant  Value=ptosim.rodLength
  Divide : Product  Inputs=*/
  Divide1 : Product  Inputs=*/
  Gain : Gain  Gain=-1
  Product : Product
  Product1 : Product
  Sqrt : Sqrt  SaturateOnIntegerOverflow=on
  Square : Math  Operator=square  SignedPower=on  SaturateOnIntegerOverflow=on
  Trigonometric Function : Trigonometry  Operator=cos
  Trigonometric Function1 : Trigonometry  Operator=cos
  cos_gamma : Outport
  sin_gamma : Outport  Port=2
  wires:
  Gain/1 -> cos_gamma/1
  Sqrt/1 -> Gain/1
  Constant4/1 -> Add/2
  Constant/1 -> Add2/1
  Constant5/1 -> Divide/2
  Divide/1 -> Square/1
  Trigonometric Function/1 -> Product/1
  Constant2/1 -> Product/2
  Product/1 -> Add/1
  Square/1 -> Add2/2
  angPos/1 -> Trigonometric Function/1, Trigonometric Function1/1
  Add2/1 -> Sqrt/1
  Add/1 -> Divide/1
  Constant6/1 -> Divide1/2
  Trigonometric Function1/1 -> Product1/1
  Constant1/1 -> Product1/2
  Product1/1 -> Add1/1
  Constant3/1 -> Add1/2
  Add1/1 -> Divide1/1
  Divide1/1 -> sin_gamma/1

== system Merged_Model/Osmo-Sim/Rotary to Linear Crank/Angular to Linear Position/Initial Distance btw flap joint & crank joint along x-axis ==
  Add3 : Sum  Inputs=+-
  Add4 : Sum  Inputs=+-
  Constant1 : Constant  Value=ptosim.rodLength
  Constant5 : Constant  Value=ptosim.crank
  Constant6 : Constant  Value=ptosim.offset
  Math Function2 : Math  Operator=square  SignedPower=on  SaturateOnIntegerOverflow=on
  Math Function3 : Math  Operator=square  SignedPower=on  SaturateOnIntegerOverflow=on
  Sqrt1 : Sqrt  SaturateOnIntegerOverflow=on
  d : Outport
  wires:
  Sqrt1/1 -> d/1
  Math Function2/1 -> Add3/1
  Math Function3/1 -> Add3/2
  Add4/1 -> Math Function3/1
  Constant6/1 -> Add4/2
  Constant5/1 -> Add4/1
  Constant1/1 -> Math Function2/1
  Add3/1 -> Sqrt1/1

== matlab function Merged_Model/Osmo-Sim/BRO/Iteration Function ==
  data: pi output; velo output; Q_p output; J_w_inst output; C_f input; C_b input; V_active input; V_dot_active output; p_b output; p_f output; C_dot_f output; C_dot_b output; n_shaft input; P_cp output; torque_hp output; V_D_hpp parameter; eta_cp parameter; n_par parameter; n_ser parameter; L_mem parameter; A_mem parameter; V_mem parameter; A_w parameter; thick parameter; nu parameter; D parameter; Sc parameter; b parameter; rho_f parameter; eta_hp parameter; Q_cp parameter; A_p parameter
function [pi,velo, Q_p, J_w_inst, V_dot_active, p_b, p_f, C_dot_f, C_dot_b, P_cp, torque_hp] = Iteration_Function(C_f, C_b, V_active, n_shaft, V_D_hpp, eta_cp, n_par, n_ser, L_mem, A_mem, V_mem, A_w, thick, nu, D, Sc, b, rho_f, eta_hp, Q_cp, A_p)
%% CONTROL EFFORT

%% Pump Flow Rate Conversion
Q_hp = n_shaft * V_D_hpp;              %flow rate of HPP (assuming same shaft speed as HM) [m^3/s]

%% Flow Rates and Piston Velocity
Q_p = Q_hp;                        %Permeate flow rate [m^3/s]
Q_b = Q_cp;                        %Brine flow rate [m^3/s]
Q_f = Q_hp + Q_b;                  %Feed flow rate [m^3/s]
V_dot_active = Q_b - Q_f;          %Volumetric flow rate through the tank

velo = -(V_dot_active)/A_p;        %velocity of piston [m/s]

%% Salinity Dynamics 2
D_h = 2 * thick;
C_dot_f = (-Q_f * C_f + Q_b * C_b - C_f*V_dot_active)/V_active; 
C_dot_b = 2*(Q_f * C_f - Q_b * C_b)/(V_mem * n_par * n_ser) - C_dot_f;
Q_avg = (0.5/(n_par))*(Q_f + Q_b);              %Average flow rate on feed side [m^3/s]
u_avg = Q_avg*2*L_mem/(thick*A_mem);                      %Average velocity on feed side [m/s]
Re = u_avg * thick / nu;                                      %Reynolds number                     
f = 3.23*Re^-0.3;                                       %friction factor
p_drop = n_ser*f*L_mem*rho_f*u_avg^2/(2*D_h);                 %Pressure drop across all membrane modules [Pa]


J_w_inst = Q_p/(A_mem*n_ser*n_par);                         %instantaneous flux [m/s]
Sh = .20*(Re^.57*Sc^.4);                                %Sherwood number  https://www.sciencedirect.com/science/article/pii/S0011916420313035?via%3Dihub
k = Sh*D/D_h;                                           %Mass transfer coefficient [m/s]
C_mem_avg = 0.5*(C_f+C_b);                                %Average bulk salinity on feed side [g/kg]

pi = b*C_mem_avg*exp(J_w_inst/k);                              %Feed side osmotic pressure [Pa]
p_f = J_w_inst/A_w + pi + p_drop/2;                                    %hi p pump pressure [Pa] ****************  
p_b = p_f - p_drop;                                     % pressure at circ pump inlet (Pa)

%% Torque and Power Calculation
% P_hp = Q_hp*p_in*1e5/eta_hp;            %high pressure pump power consumption [W]
P_cp = Q_cp*p_drop/eta_cp;          %circulation pump power consumption [W]
torque_hp = -(V_D_hpp * p_f) /(eta_hp*2*3.14159);        %torque generated by HPP (NOTE: opposite sign as n_shaft!)
